simulink model "linear_model"  (R2020a)
settings: Solver=ode45  StartTime=0.0  StopTime=simulation_time  FixedStep=sample_time  RelTol=1e-3
values from neighbouring files (symbols this model uses):
  C = [0 mw 0 0             -1        0         0 1;      0 0  0 0             0         1         1 0;      0 mp 0 -mp*L*cos(x3) 1         0         0 0;      0 0  0 mp*L*sin(x3)  0         -1        0 0;      0 0  0 0             0         0         0 Rw;      0 0  0 0             L*cos(x3) L*sin(x3) 0 0;      1 0  0 0             0         0         0 0 ... (first row only)    [balance_ode.m]    (also in lab06.m = eye(4))
  D = zeros(4,1)    [lab06.m]
  K = lqr(A, B, Q, R)    [lab06.m]
  sample_time = 0.03    [lab06.m]
  x0 = [0; 0; deg2rad(2); 0]    [lab06.m]
undefined symbols (not defined in the file or in its folder): A, B
settings Model: Creator=donelp  LastModifiedBy=donelp
settings DataIOCC: SaveOutput=off  SignalLogging=off  DSMLogging=off  SaveTime=off  ReturnWorkspaceOutputs=off

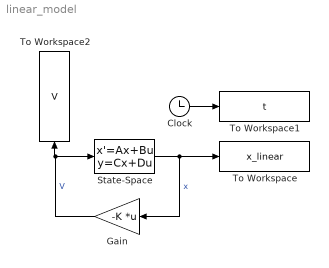
== system linear_model ==
  Clock : Clock
  Gain : Gain  Gain=-K  Multiplication=Matrix(K*u)
  State-Space : StateSpace  A=A  B=B  C=C  D=D  InitialCondition=x0
  To Workspace : ToWorkspace  VariableName=x_linear  SampleTime=sample_time
      settings: Save2DSignal=2-D array (concatenate along first dimension)
  To Workspace1 : ToWorkspace  VariableName=t  SampleTime=sample_time
      settings: Save2DSignal=2-D array (concatenate along first dimension)
  To Workspace2 : ToWorkspace  VariableName=V  SampleTime=sample_time
      settings: Save2DSignal=2-D array (concatenate along first dimension)
  wires:
  Gain/1 -> State-Space/1, To Workspace2/1  "V"
  State-Space/1 -> Gain/1, To Workspace/1  "x"
  Clock/1 -> To Workspace1/1
